simulink model "sistemacomcontrole"  (Simulink 4.00)
settings: Solver=ode45  StartTime=0.0  StopTime=3  MaxStep=0.00001  RelTol=1e-3
settings Model: LastModifiedBy=Gui

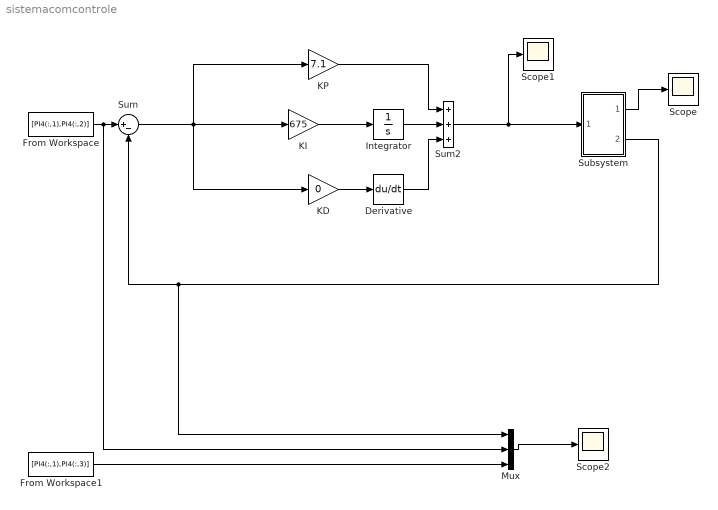
== system sistemacomcontrole ==
  Derivative : Derivative
  From Workspace : FromWorkspace  VariableName=[PI4(:,1),PI4(:,2)]  SampleTime=0  OutputAfterFinalValue=Extrapolation
  From Workspace1 : FromWorkspace  VariableName=[PI4(:,1),PI4(:,3)]  SampleTime=0  OutputAfterFinalValue=Extrapolation
  Integrator : Integrator  ExternalReset=none  InitialConditionSource=internal  InitialCondition=0  LimitOutput=off  UpperSaturationLimit=inf  LowerSaturationLimit=-inf  ShowSaturationPort=off  ShowStatePort=off  AbsoluteTolerance=auto
  KD : Gain  Gain=0  Multiplication=Element-wise(K.*u)  SaturateOnIntegerOverflow=on
  KI : Gain  Gain=675  Multiplication=Element-wise(K.*u)  SaturateOnIntegerOverflow=on
  KP : Gain  Gain=7.1  Multiplication=Element-wise(K.*u)  SaturateOnIntegerOverflow=on
  Mux : Mux  Inputs=3
  Scope : Scope
      settings: TimeRange=auto  YMin=-5  YMax=5  SaveToWorkspace=off  SaveName=ScopeData  MaxDataPoints=5000
  Scope1 : Scope
      settings: TimeRange=0.05  YMin=-0.5  YMax=4.5  SaveToWorkspace=off  MaxDataPoints=5000
  Scope2 : Scope
      settings: TimeRange=0.05  YMin=0.5  YMax=7  SaveToWorkspace=off  SaveName=ScopeData2  MaxDataPoints=5000
  Subsystem : Subsystem
      settings: RTWFcnNameOpts=Auto  RTWFileNameOpts=Auto
  Sum : Sum  Inputs=|+-  SaturateOnIntegerOverflow=on
  Sum2 : Sum  Inputs=+++  SaturateOnIntegerOverflow=on
  wires:
  KI/1 -> Integrator/1
  KP/1 -> Sum2/1
  Derivative/1 -> Sum2/3
  KD/1 -> Derivative/1
  Sum2/1 -> Subsystem/1(In1), Scope1/1
  Integrator/1 -> Sum2/2
  Sum/1 -> KI/1, KD/1, KP/1
  Mux/1 -> Scope2/1
  Subsystem/2(Out2) -> Sum/2, Mux/1
  Subsystem/1(Out1) -> Scope/1
  From Workspace/1 -> Sum/1, Mux/2
  From Workspace1/1 -> Mux/3

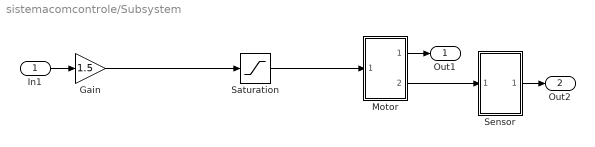
== system sistemacomcontrole/Subsystem ==
  In1 : Inport  Port=1  LatchInput=off
  Gain : Gain  Gain=1.5  Multiplication=Element-wise(K.*u)  SaturateOnIntegerOverflow=on
  Motor : Subsystem
      settings: RTWFcnNameOpts=Auto  RTWFileNameOpts=Auto
  Saturation : Saturate  UpperLimit=13.5  LowerLimit=-13.99  LinearizeAsGain=on
  Sensor : Subsystem
      settings: RTWFcnNameOpts=Auto  RTWFileNameOpts=Auto
  Out1 : Outport  Port=1
  Out2 : Outport  Port=2
  wires:
  Motor/2(Out2) -> Sensor/1(In1)
  Motor/1(Out1) -> Out1/1
  In1/1 -> Gain/1
  Sensor/1(Out1) -> Out2/1
  Gain/1 -> Saturation/1
  Saturation/1 -> Motor/1(In1)

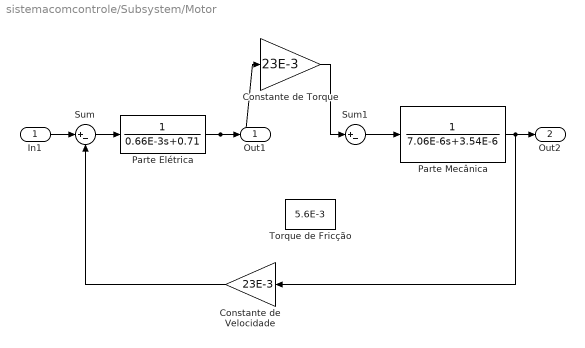
== system sistemacomcontrole/Subsystem/Motor ==
  In1 : Inport  Port=1  LatchInput=off
  Constante de Torque : Gain  Gain=23E-3  Multiplication=Element-wise(K.*u)  SaturateOnIntegerOverflow=on
  Constante de Velocidade : Gain  Orientation=left  Gain=23E-3  Multiplication=Element-wise(K.*u)  SaturateOnIntegerOverflow=on
  Parte Elétrica : TransferFcn  Numerator=[1]  Denominator=[0.66E-3 0.71]  AbsoluteTolerance=auto  Realization=auto
  Parte Mecânica : TransferFcn  Numerator=[1]  Denominator=[7.06E-6 3.54E-6]  AbsoluteTolerance=auto  Realization=auto
  Sum : Sum  Inputs=|+-  SaturateOnIntegerOverflow=on
  Sum1 : Sum  Inputs=|+-  SaturateOnIntegerOverflow=on
  Torque de Fricção : Constant  Value=5.6E-3
  Out1 : Outport  Port=1
  Out2 : Outport  Port=2
  wires:
  Sum/1 -> Parte Elétrica/1
  Parte Elétrica/1 -> Constante de Torque/1, Out1/1
  Parte Mecânica/1 -> Constante de Velocidade/1, Out2/1
  Constante de Velocidade/1 -> Sum/2
  Constante de Torque/1 -> Sum1/1
  Sum1/1 -> Parte Mecânica/1
  In1/1 -> Sum/1

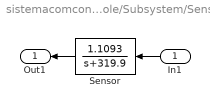
== system sistemacomcontrole/Subsystem/Sensor ==
  In1 : Inport  Orientation=left  Port=1  LatchInput=off
  "Sensor " : TransferFcn  Orientation=left  Numerator=[1.1093]  Denominator=[1 319.9]  AbsoluteTolerance=auto  Realization=auto
  Out1 : Outport  Orientation=left  Port=1
  wires:
  "Sensor "/1 -> Out1/1
  In1/1 -> "Sensor "/1
